simulink model "RCAM_Simulation"  (R2020b)
settings: Solver=VariableStepAuto  StartTime=0.0  StopTime=tStop  FixedStep=0.1  MaxStep=1  RelTol=1e-3
values from neighbouring files (symbols this model uses):
  geo0 = [deg2rad(-157.9251) deg2rad(21.32451) h]'    [TrimAndLinearize.m]
  p0 = [0 0 0]'    [TrimAndLinearize.m]
  u0 = [0;0;0;0.0079;0.0079]    [TrimAndLinearize.m]
  x = x_trimmed    [TrimAndLinearize.m]
undefined symbols (not defined in the file or in its folder): body2NED_velocity, curvatures, geos, RCAM
libraries: aerolibfltsims x2, vrlib x1
settings Model: Creator=SAMAD AeroDesk  LastModifiedBy=apple-ios
settings SolverCC: InitialStep=0.1
settings SFSimCC: CustomCodeUndefinedFunction=UseInterfaceOnly

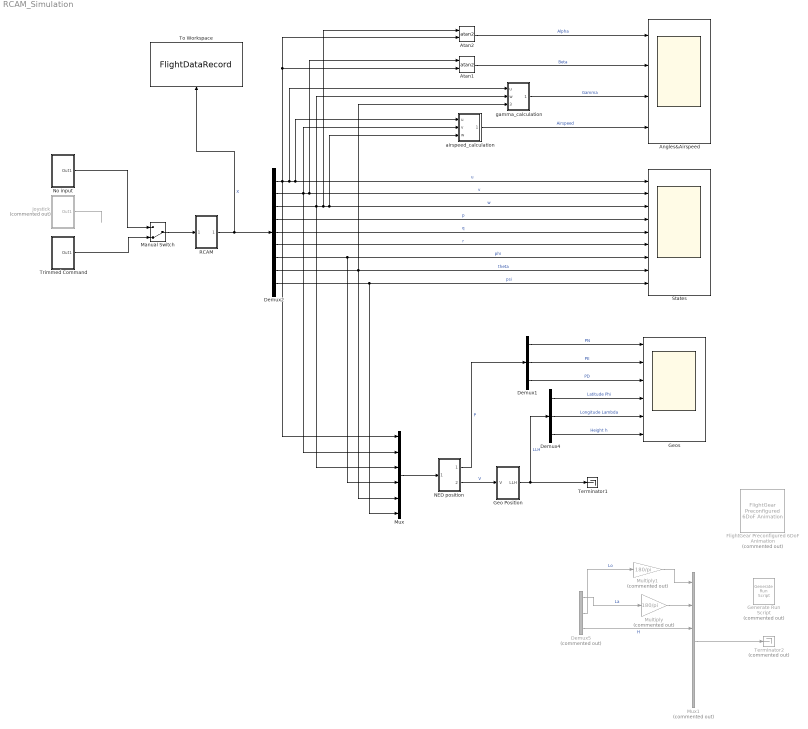
== system RCAM_Simulation ==
  Angles&Airspeed : Scope  NumInputPorts=4
  Atan1 : Trigonometry  Operator=atan2
  Atan2 : Trigonometry  Operator=atan2
  Demux1 : Demux  Outputs=3
  Demux2 : Demux  Outputs=9
  Demux4 : Demux  Outputs=3
  Demux5 : Demux  Commented=on  Outputs=3
  FlightGear Preconfigured 6DoF Animation : aerolibfltsims/FlightGear Preconfigured 6DoF Animation  Commented=on  xFlightGearVersion=v2019.1  DestinationIpAddress=127.0.0.1  DestinationPort=5502  SampleTime=1/30  packetVersion=24
  Generate Run Script : aerolibfltsims/Generate Run Script  Commented=on  Architecture=Win64  dataFlow=Send  GeometryModelName=c172p  AirportId=KSFO  RunwayId=10L  InitialAltitude=7224  InitialHeading=113  OffsetDistance=4.72  OffsetAzimuth=0  InstallScenery=off  DisableShaders=on  OriginAddress=127.0.0.1  DestinationPort=5502  OriginPort=5505  LocalAddress=127.0.0.1  OutputFileName=runfg.bat  FlightGearBaseDirectory=D:\FlightGear 2020.3.6
  Geo Position : Subsystem
  Geos : Scope  NumInputPorts=6
  Joystick : Subsystem  Commented=on
  Manual Switch : ManualSwitch  CurrentSetting=0
  Multiply : Gain  Commented=on  Gain=180/pi
  Multiply1 : Gain  Commented=on  Gain=180/pi
  Mux : Mux  Inputs=6
  Mux1 : Mux  Commented=on  Inputs=6
  NED position : Subsystem
  No input : Subsystem
  RCAM : Subsystem
  States : Scope  NumInputPorts=9
  Terminator1 : Terminator
  Terminator2 : Terminator  Commented=on
  To Workspace : ToWorkspace  VariableName=FlightDataRecord  SaveFormat=Structure With Time  SampleTime=-1
      settings: Save2DSignal=2-D array (concatenate along first dimension)
  Trimmed Command : Subsystem
  airspeed_calculation : Subsystem
  gamma_calculation : Subsystem
  wires:
  Demux2/9 -> Mux/6, States/9  "psi"
  Demux2/4 -> States/4  "p"
  Mux1/1 -> Terminator2/1
  Demux4/1 -> Geos/4  "Latitude Phi"
  Demux5/3 -> Mux1/3  "H"
  Multiply/1 -> Mux1/2
  Demux4/3 -> Geos/6  "Height h"
  Multiply1/1 -> Mux1/1
  Demux4/2 -> Geos/5  "Longitude Lambda"
  Demux5/1 -> Multiply/1  "La"
  Demux5/2 -> Multiply1/1  "Lo"
  RCAM/1(Out1) -> To Workspace/1, Demux2/1  "X"
  NED position/2(Output) -> Geo Position/1(V)  "V"
  Demux1/2 -> Geos/2  "PE"
  Demux1/1 -> Geos/1  "PN"
  Demux2/6 -> States/6  "r"
  Mux/1 -> NED position/1(In1)
  Demux2/7 -> Mux/4, States/7  "phi"
  Demux2/5 -> States/5  "q"
  Demux1/3 -> Geos/3  "PD"
  NED position/1(Out1) -> Demux1/1  "P"
  Geo Position/1(LLH) -> Terminator1/1, Demux4/1  "LLH"
  Joystick/1(Out1) -> ?
  Trimmed Command/1(Out1) -> Manual Switch/2
  Manual Switch/1 -> RCAM/1(In1)
  No input/1(Out1) -> Manual Switch/1
  Atan1/1 -> Angles&Airspeed/2  "Beta"
  Atan2/1 -> Angles&Airspeed/1  "Alpha"
  ? -> Demux5/1
  gamma_calculation/1(Out1) -> Angles&Airspeed/3  "Gamma"
  Demux2/1 -> States/1, airspeed_calculation/1(u), gamma_calculation/1(u), Atan1/2, Atan2/2, Mux/1  "u"
  Demux2/8 -> States/8, gamma_calculation/3(theta), Mux/5  "theta"
  Demux2/3 -> States/3, airspeed_calculation/3(w), Atan2/1, Mux/3, gamma_calculation/2(w)  "w"
  Demux2/2 -> Mux/2, States/2, Atan1/1, airspeed_calculation/2(v)  "v"
  airspeed_calculation/1(Output) -> Angles&Airspeed/4  "Airspeed"

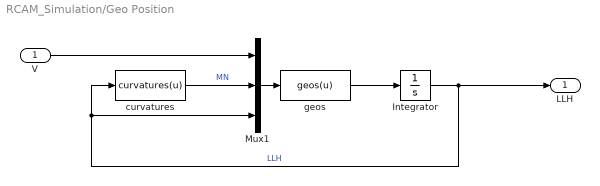
== system RCAM_Simulation/Geo Position ==
  V : Inport
  Integrator : Integrator  InitialCondition=geo0
  Mux1 : Mux  Inputs=3
  curvatures : MATLABFcn  MATLABFcn=curvatures(u)
  geos : MATLABFcn  MATLABFcn=geos(u)
  LLH : Outport
  wires:
  Mux1/1 -> geos/1
  V/1 -> Mux1/1
  geos/1 -> Integrator/1
  Integrator/1 -> Mux1/3, curvatures/1, LLH/1  "LLH"
  curvatures/1 -> Mux1/2  "MN"

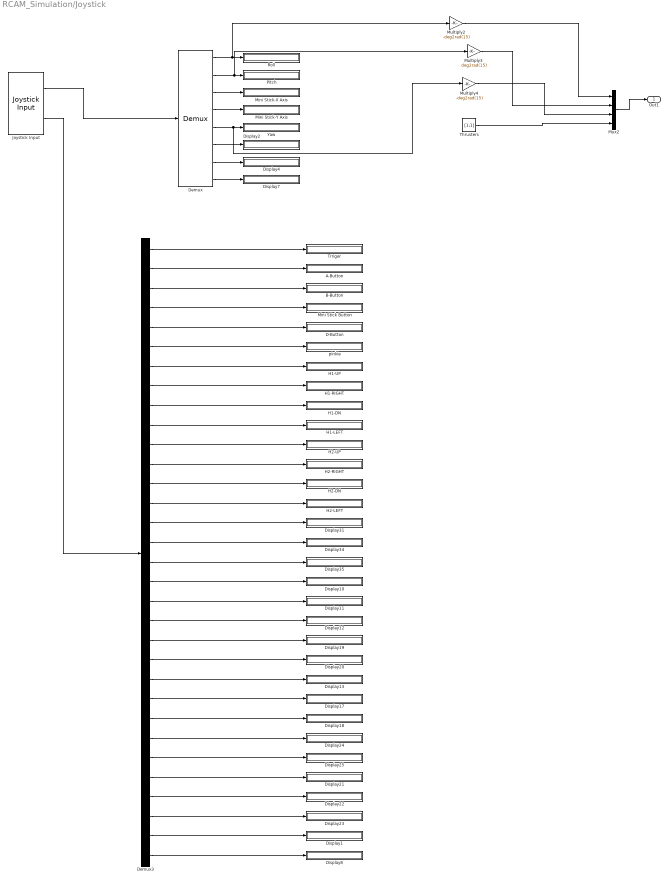
== system RCAM_Simulation/Joystick ==
  A-Button : Display
  B-Button : Display
  D-Button : Display
  Demux : Demux  Outputs=8
      settings: DisplayOption=none
  Demux3 : Demux  Outputs=32
  Display{1..2,4,7..8,10..13,17..25,31,34..35} (21 alike) : Display
  H1-DN : Display
  H1-LEFT : Display
  H1-RIGHT : Display
  H1-UP : Display
  H2-DN : Display
  H2-LEFT : Display
  H2-RIGHT : Display
  H2-UP : Display
  Joystick Input : vrlib/Joystick Input  joyid=2  adjustports=off  forcefeed=off
      settings: AttributesFormatString=(Joystick ID and Axes\nmust be set properly!)
  Mini Stick Button : Display
  Mini Stick-X Axis : Display
  Mini Stick-Y Axis : Display
  Multiply2 : Gain  Gain=-deg2rad(15)
  Multiply3 : Gain  Gain=deg2rad(15)
  Multiply4 : Gain  Gain=-deg2rad(15)
  Mux2 : Mux
  Pitch : Display
  Roll : Display
  Thrusters : Constant  Value=[1;1]
  Trriger : Display
  Yaw : Display
  pinkie : Display
  Out1 : Outport
  wires:
  Demux3/30 -> Display23/1
  Demux/2 -> Multiply3/1, Pitch/1
  Demux3/25 -> Display18/1
  Multiply3/1 -> Mux2/2
  Demux3/10 -> H1-LEFT/1
  Thrusters/1 -> Mux2/4
  Demux3/15 -> Display31/1
  Multiply4/1 -> Mux2/3
  Joystick Input/1 -> Demux/1
  Demux3/27 -> Display25/1
  Demux3/6 -> pinkie/1
  Demux/3 -> Mini Stick-X Axis/1
  Demux3/28 -> Display21/1
  Demux3/31 -> Display1/1
  Demux3/24 -> Display17/1
  Demux3/11 -> H2-UP/1
  Multiply2/1 -> Mux2/1
  Demux3/1 -> Trriger/1
  Demux3/18 -> Display10/1
  Demux3/7 -> H1-UP/1
  Demux3/16 -> Display34/1
  Demux3/32 -> Display8/1
  Demux3/19 -> Display11/1
  Demux3/17 -> Display35/1
  Demux/5 -> Multiply4/1, Yaw/1
  Demux3/8 -> H1-RIGHT/1
  Demux3/13 -> H2-DN/1
  Demux3/3 -> B-Button/1
  Demux3/22 -> Display20/1
  Demux3/14 -> H2-LEFT/1
  Joystick Input/2 -> Demux3/1
  Demux3/4 -> Mini Stick Button/1
  Demux/4 -> Mini Stick-Y Axis/1
  Demux/8 -> Display7/1
  Demux3/5 -> D-Button/1
  Demux3/20 -> Display12/1
  Demux3/23 -> Display13/1
  Demux3/9 -> H1-DN/1
  Demux/7 -> Display4/1
  Demux3/26 -> Display24/1
  Demux/1 -> Multiply2/1, Roll/1
  Demux3/29 -> Display22/1
  Demux3/21 -> Display19/1
  Demux3/2 -> A-Button/1
  Mux2/1 -> Out1/1
  Demux3/12 -> H2-RIGHT/1
  Demux/6 -> Display2/1

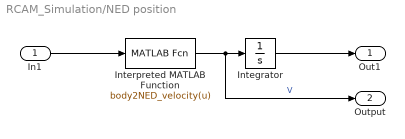
== system RCAM_Simulation/NED position ==
  In1 : Inport
  Integrator : Integrator  InitialCondition=p0
  Interpreted MATLAB Function : MATLABFcn  MATLABFcn=body2NED_velocity(u)
  Out1 : Outport
  Output : Outport  Port=2
  wires:
  In1/1 -> Interpreted MATLAB Function/1
  Integrator/1 -> Out1/1
  Interpreted MATLAB Function/1 -> Output/1, Integrator/1  "V"

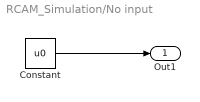
== system RCAM_Simulation/No input ==
  Constant : Constant  Value=u0
  Out1 : Outport
  wires:
  Constant/1 -> Out1/1

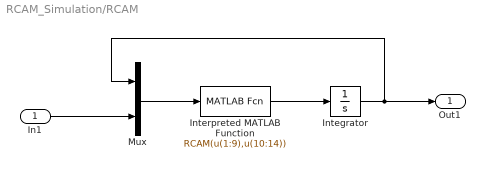
== system RCAM_Simulation/RCAM ==
  In1 : Inport
  Integrator : Integrator  InitialCondition=x
  Interpreted MATLAB Function : MATLABFcn  MATLABFcn=RCAM(u(1:9),u(10:14))
  Mux : Mux  Inputs=2
  Out1 : Outport
  wires:
  In1/1 -> Mux/2
  Mux/1 -> Interpreted MATLAB Function/1
  Integrator/1 -> Out1/1, Mux/1
  Interpreted MATLAB Function/1 -> Integrator/1

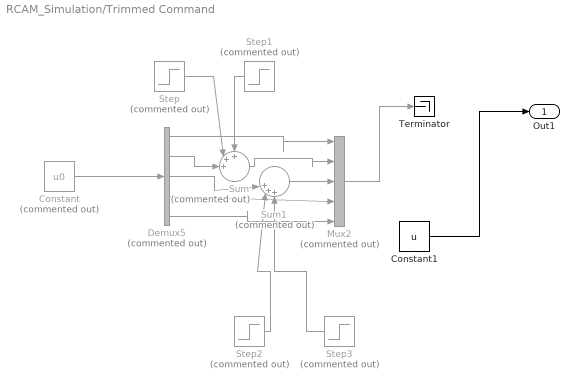
== system RCAM_Simulation/Trimmed Command ==
  Constant : Constant  Commented=on  Value=u0
  Constant1 : Constant  Value=u
  Demux5 : Demux  Commented=on  Outputs=5
  Mux2 : Mux  Commented=on  Inputs=5
  Step : Step  Commented=on  Time=3  After=-0.1  SampleTime=0
  Step1 : Step  Commented=on  Time=4  After=0.1  SampleTime=0
  Step2 : Step  Commented=on  Time=8  After=0.3  SampleTime=0
  Step3 : Step  Commented=on  Time=9  After=-0.3  SampleTime=0
  Sum : Sum  Commented=on  Inputs=+++||
  Sum1 : Sum  Commented=on  Inputs=|||+++
  Terminator : Terminator
  Out1 : Outport
  wires:
  Constant/1 -> Demux5/1
  Step1/1 -> Sum/1
  Demux5/3 -> Sum1/1
  Sum/1 -> Mux2/2
  Step2/1 -> Sum1/2
  Sum1/1 -> Mux2/3
  Demux5/5 -> Mux2/5
  Demux5/2 -> Sum/3
  Demux5/4 -> Mux2/4
  Step3/1 -> Sum1/3
  Step/1 -> Sum/2
  Demux5/1 -> Mux2/1
  Mux2/1 -> Terminator/1
  Constant1/1 -> Out1/1

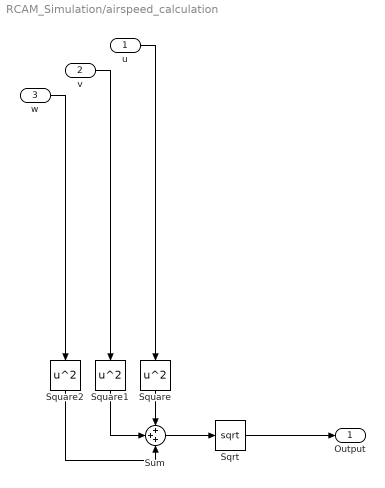
== system RCAM_Simulation/airspeed_calculation ==
  u : Inport
  v : Inport  Port=2
  w : Inport  Port=3
  Sqrt : Sqrt  SaturateOnIntegerOverflow=on
  Square : Math  Operator=square  SaturateOnIntegerOverflow=on
  Square1 : Math  Operator=square  SaturateOnIntegerOverflow=on
  Square2 : Math  Operator=square  SaturateOnIntegerOverflow=on
  Sum : Sum  Inputs=3
  Output : Outport
  wires:
  w/1 -> Square2/1
  Square/1 -> Sum/1
  Square1/1 -> Sum/2
  u/1 -> Square/1
  Sqrt/1 -> Output/1
  Sum/1 -> Sqrt/1
  v/1 -> Square1/1
  Square2/1 -> Sum/3

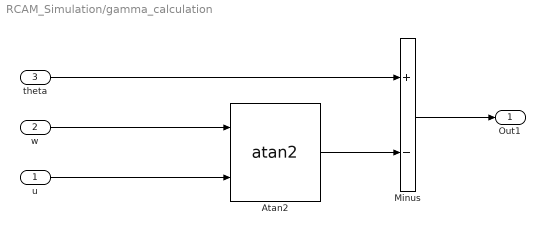
== system RCAM_Simulation/gamma_calculation ==
  u : Inport
  w : Inport  Port=2
  theta : Inport  Port=3
  Atan2 : Trigonometry  Operator=atan2
  Minus : Sum  Inputs=+-
  Out1 : Outport
  wires:
  w/1 -> Atan2/1
  Minus/1 -> Out1/1
  u/1 -> Atan2/2
  theta/1 -> Minus/1
  Atan2/1 -> Minus/2
